simulink model "lab1_parte2"  (R2022a)
settings: Solver=VariableStepAuto  StartTime=0.0  StopTime=10.0  RelTol=1e-3
settings Model: Creator=Paulo  LastModifiedBy=Paulo

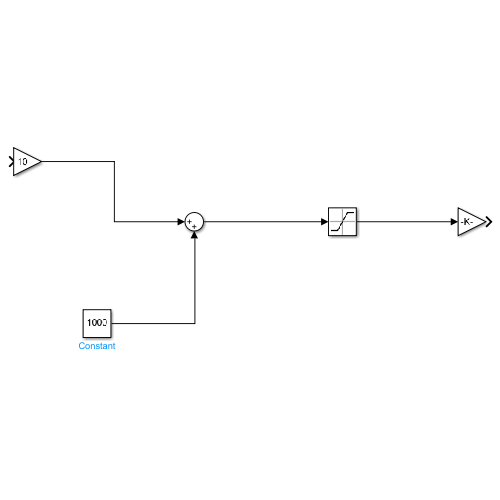
[thumbnail: Simulink's stored preview of the top-level diagram]
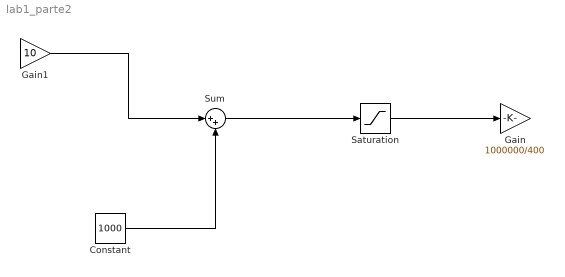
== system lab1_parte2 ==
  Constant : Constant  Value=1000
  Gain : Gain  Gain=1000000/400
  Gain1 : Gain  Gain=10
  Saturation : Saturate  UpperLimit=2000  LowerLimit=1000
  Sum : Sum  Inputs=|++
  wires:
  Saturation/1 -> Gain/1
  Gain1/1 -> Sum/1
  Sum/1 -> Saturation/1
  Constant/1 -> Sum/2
